simulink model "udp_control_system"  (R2021b)
settings: Solver=FixedStepDiscrete  StartTime=0.0  StopTime=inf  FixedStep=0.05  RelTol=1e-3
libraries: instrumentlib x2
settings Model: xpc_rtwmakecfg_data=_xpciplib__xpcetherlib__xpcether8255xlib__xpcetherGbElib__xpcnblib_  Creator=Barti  LastModifiedBy=adria
settings SolverCC: AlgebraicLoopSolver=TrustRegion
settings DataIOCC: ReturnWorkspaceOutputs=off
settings DebuggingCC: SFMachineParentedDataDiag=warning  ArithmeticOperatorsInVariantConditions=warning
settings SFSimCC: SimUseLocalCustomCode=off  CustomCodeUndefinedFunction=UseInterfaceOnly
settings RTWCC: RTWUseLocalCustomCode=off
settings CodeAppCC: StateflowObjectComments=on

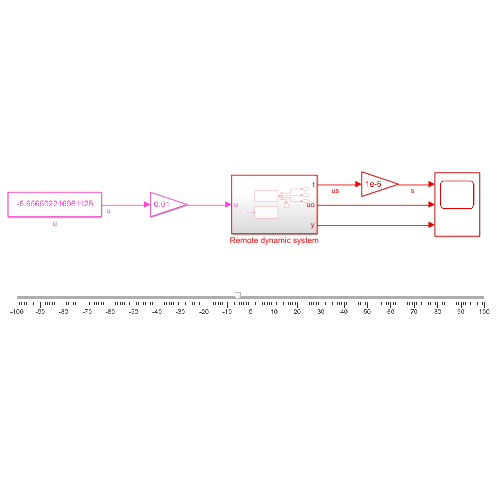
[thumbnail: Simulink's stored preview of the top-level diagram]
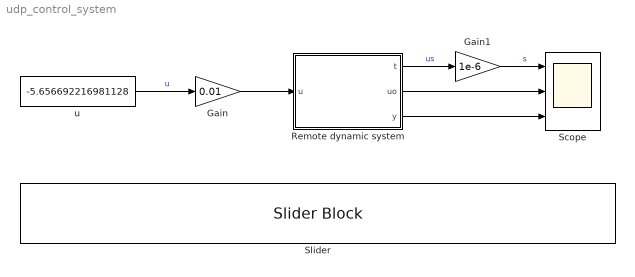
== system udp_control_system ==
  Gain : Gain  Gain=0.01
  Gain1 : Gain  Gain=1e-6
  Remote dynamic system : Subsystem
  Scope : Scope  NumInputPorts=3
  Slider : SliderBlock  LabelPosition=Hide  ScaleMin=-100  TickInterval=10
  u : Constant  Value=-5.656692216981128  OutDataTypeStr=single
  wires:
  u/1 -> Gain/1  "u"
  Gain/1 -> Remote dynamic system/1(u)
  Remote dynamic system/2(uo) -> Scope/2
  Remote dynamic system/3(y) -> Scope/3
  Gain1/1 -> Scope/1  "s"
  Remote dynamic system/1(t) -> Gain1/1  "us"

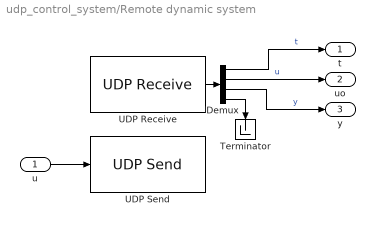
== system udp_control_system/Remote dynamic system ==
  u : Inport
  Demux : Demux
  Terminator : Terminator
  UDP Receive : instrumentlib/UDP Receive  Host=172.27.229.191  Port=20001  LocalPort=25000  EnablePortSharing=off  GetLatestData=off  DataSize="[1  4]"  DataType=single  ASCIIFormatting=%d  Terminator=LF  ByteOrder=LittleEndian  EnableBlockingMode=on  Timeout=10  SampleTime=0.05  LocalAddress=172.27.224.1
  UDP Send : instrumentlib/UDP Send  Host=172.27.229.191  Port=20002  LocalPort=25001  EnablePortSharing=off  ByteOrder=LittleEndian  OutputDatagramPacketSize=512  EnableBlockingMode=on  LocalAddress=172.27.224.1
  t : Outport
  uo : Outport  Port=2
  y : Outport  Port=3
  wires:
  UDP Receive/1 -> Demux/1
  Demux/4 -> Terminator/1
  Demux/2 -> uo/1  "u"
  Demux/3 -> y/1  "y"
  Demux/1 -> t/1  "t"
  u/1 -> UDP Send/1
